simulink model "thrust_curve_import_test"  (R2014a)
settings: Solver=ode45  StartTime=0.0  StopTime=10.0  RelTol=1e-3
libraries: simulink x1
settings Model: Creator=scorpii  LastModifiedBy=scorpii

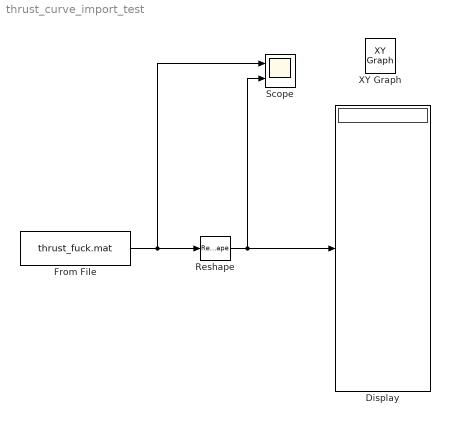
== system thrust_curve_import_test ==
  Display : Display
  From File : FromFile  FileName=thrust_fuck.mat  SampleTime=0
  Reshape : Reshape
  Scope : Scope  NumInputPorts=2
      settings: YMin=0~0  YMax=2500~2500
  XY Graph : simulink/Sinks/XY Graph  xmin=-1  xmax=1  ymin=-1  ymax=1  st=-1
  wires:
  Reshape/1 -> Scope/2, Display/1
  From File/1 -> Scope/1, Reshape/1
